simulink model "wah"  (R2017b)
settings: Solver=ode45  StartTime=0.0  StopTime=10.0  MaxStep=0.01  RelTol=1e-3
settings Model: Creator=ba39216  LastModifiedBy=ba39216

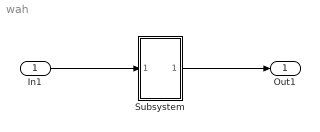
== system wah ==
  In1 : Inport
  Subsystem : Subsystem  mask{m=2, l=1, g=9.81, k=2}
      mask prompts: m "masa"; l "długość wahadła"; g "przyspieszenie ziemskie"; k "współczynik tłumienia"
  Out1 : Outport
  wires:
  In1/1 -> Subsystem/1(In1)
  Subsystem/1(Out1) -> Out1/1

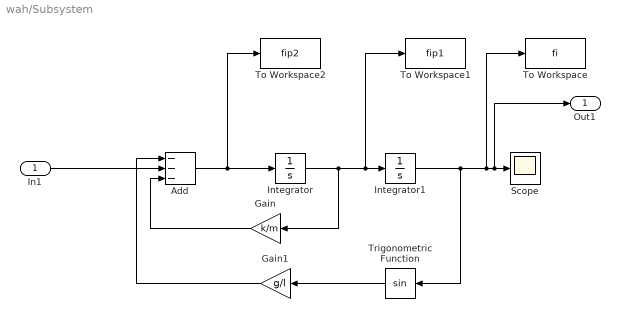
== system wah/Subsystem ==
  In1 : Inport
  Add : Sum  Inputs=---
  Gain : Gain  Gain=k/m
  Gain1 : Gain  Gain=g/l
  Integrator : Integrator
  Integrator1 : Integrator  InitialCondition=pi/2
  Scope : Scope
  To Workspace : ToWorkspace  VariableName=fi  SampleTime=-1
  To Workspace1 : ToWorkspace  VariableName=fip1  SampleTime=-1
  To Workspace2 : ToWorkspace  VariableName=fip2  SampleTime=-1
  Trigonometric Function : Trigonometry
  Out1 : Outport
  wires:
  Integrator1/1 -> Trigonometric Function/1, To Workspace/1, Out1/1, Scope/1
  Gain1/1 -> Add/1
  Integrator/1 -> Gain/1, To Workspace1/1, Integrator1/1
  Gain/1 -> Add/3
  Add/1 -> To Workspace2/1, Integrator/1
  Trigonometric Function/1 -> Gain1/1
  In1/1 -> Add/2
